simulink model "TestFLOWchart"  (Simulink 7.8)
settings: Solver=ode45  StartTime=0.0  StopTime=10.0  RelTol=1e-3
settings Model: Creator=ASL  LastModifiedBy=ASL

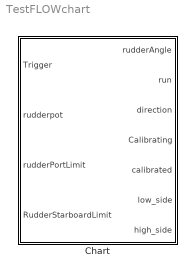
== system TestFLOWchart ==
  Chart : Stateflow chart  TreatAsAtomicUnit=on

== stateflow chart Chart ==
  state %Waiting For Trigger
    entry:   low_side = int32(-1);
    high_side = int32(-1);
    calibrated = false;
  state %Drive towards Center
    entry: direction = false;
    exit: run =false;
    exit: calibrating=false
  state %Drive towards port
    entry: direction = true;
    exit: low_side = input;
    exit: if(high_side < low_side)
    high_side = high_side +1023
    end
    exit: calibrated =true
  state %Drive towards Sb
    entry:  run = true;
    direction = false;
    calibrating = true;
    exit: high_side = input;
  %Drive towards port -> %Drive towards Center : if(rudderPortLimit)
  %Drive towards Sb -> %Drive towards port : if(RudderStarboardLimit)
  %Waiting For Trigger -> %Drive towards Sb : If(Trigger)
  (default) -> %Waiting For Trigger
  %Drive towards Center -> %Waiting For Trigger
  data: Trigger input double; rudderpot input double; rudderPortLimit input double; RudderStarboardLimit input double; rudderAngle output single; run output boolean; direction output boolean; Calibrating output boolean; calibrated output boolean; low_side output uint16; high_side output uint16
